simulink model "lab04z2_sch"  (Simulink 10.3)
settings: Solver=ode3  StartTime=0.0  StopTime=10  FixedStep=0.001  RelTol=1e-3  EnableMultiTasking=on
InitFcn:
  | % Parametry obiektu
  | R = 3;
  | L = 0.05;
  | kfi = 2.23;
  | J = 0.11;
values from neighbouring files (symbols this model uses):
  ki = 1    [lab04z1.m]
  Kx = acker(A, B, [-wc, -wc])    [lab04z1.m]
  Lo = acker(A', C', [-w0, -w0])    [lab04z1.m]
undefined symbols (not defined in the file or in its folder): regStan
settings Model: Creator=Jacek  LastModifiedBy=AgraWoodAdmin
settings DataIOCC: LimitDataPoints=on  SignalLoggingSaveFormat=Dataset
settings OptimizationCC: ExpressionDepthLimit=128
settings DebuggingCC: UnderspecifiedInitializationDetection=Simplified  MergeDetectMultiDrivingBlocksExec=error  SolverPrmCheckMsg=warning  FcnCallInpInsideContextMsg=error  StateNameClashWarn=none
settings GRTTargetCC: CombineOutputUpdateFcns=on  GRTInterface=off
settings ConfigComp: CovSFcnEnable=off

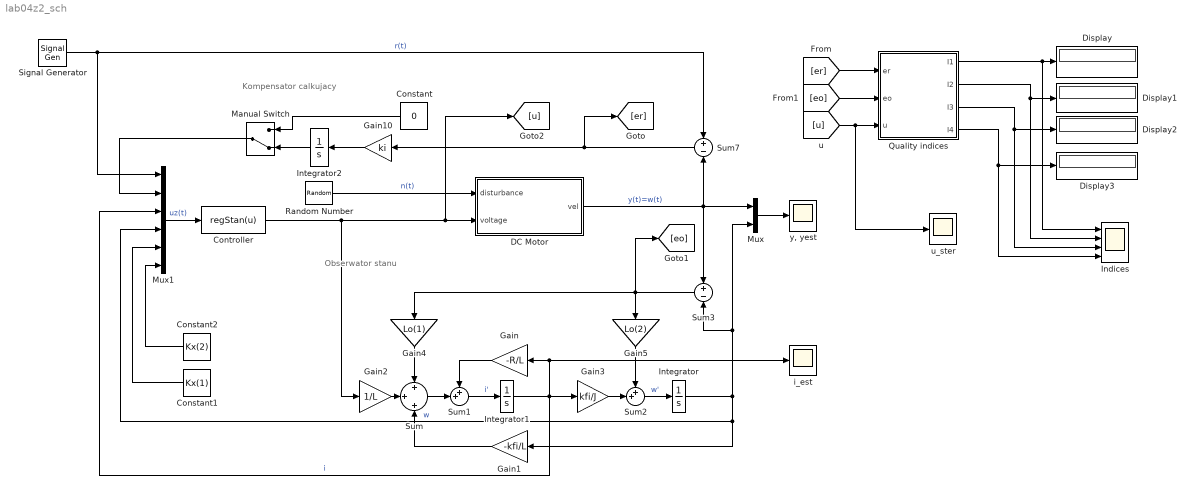
== system lab04z2_sch ==
  note: Kompensator calkujacy
  note: Obserwator stanu
  Constant : Constant  Value=0
  Constant1 : Constant  Value=Kx(1)
  Constant2 : Constant  Value=Kx(2)
  Controller : MATLABFcn  MATLABFcn=regStan(u)  OutputDimensions=1
  DC Motor : Subsystem
  Display{,1..3} (4 alike) : Display
  Gain : Gain  Gain=-R/L
  Gain1 : Gain  Gain=-kfi/L
  Gain10 : Gain  Gain=ki
  Gain2 : Gain  Gain=1/L
  Gain3 : Gain  Gain=kfi/J
  Gain4 : Gain  Gain=Lo(1)
  Gain5 : Gain  Gain=Lo(2)
  Indices : Scope  NumInputPorts=4
  Integrator : Integrator  InitialCondition=40
  Integrator1 : Integrator  InitialCondition=20
  Integrator2 : Integrator
  Manual Switch : ManualSwitch  CurrentSetting=0
  Mux : Mux  Inputs=2
  Mux1 : Mux  Inputs=6
  Quality indices : Subsystem
  Random Number : RandomNumber  Variance=10
  Signal Generator : SignalGenerator  WaveForm=square  Amplitude=200  Frequency=0.5
  Sum : Sum  Inputs=+|+|+
  Sum1 : Sum  Inputs=++|
  Sum2 : Sum  Inputs=++|
  Sum3 : Sum  Inputs=+|-
  Sum7 : Sum  Inputs=+|-
  i_est : Scope
  u_ster : Scope
  "y, yest" : Scope
  wires:
  Random Number/1 -> DC Motor/1(disturbance)  "n(t)"
  Mux1/1 -> Controller/1  "uz(t)"
  DC Motor/1(vel) -> Sum3/1, Sum7/2, Mux/1  "y(t)=w(t)"
  Gain2/1 -> Sum/2
  Sum1/1 -> Integrator1/1  "i'"
  Gain/1 -> Sum1/1
  Sum/1 -> Sum1/2
  Gain1/1 -> Sum/3
  Sum2/1 -> Integrator/1  "w'"
  Gain3/1 -> Sum2/2
  Sum3/1 -> [eo], Gain5/1, Gain4/1
  Gain5/1 -> Sum2/1
  Gain4/1 -> Sum/1
  Mux/1 -> "y, yest"/1
  Integrator/1 -> Mux1/4, Gain1/1, Sum3/2, Mux/2  "w"
  Integrator1/1 -> i_est/1, Gain/1, Mux1/3, Gain3/1  "i"
  Signal Generator/1 -> Mux1/1, Sum7/1  "r(t)"
  Integrator2/1 -> Manual Switch/2
  Sum7/1 -> [er], Gain10/1
  Gain10/1 -> Integrator2/1
  Manual Switch/1 -> Mux1/2
  Constant/1 -> Manual Switch/1
  Quality indices/4(I4) -> Indices/4, Display3/1
  Quality indices/1(I1) -> Indices/1, Display/1
  Quality indices/2(I2) -> Display1/1, Indices/2
  Quality indices/3(I3) -> Display2/1, Indices/3
  [er] -> Quality indices/1(er)
  [eo] -> Quality indices/2(eo)
  [u] -> u_ster/1, Quality indices/3(u)
  Constant2/1 -> Mux1/6
  Constant1/1 -> Mux1/5
  Controller/1 -> Gain2/1, [u], DC Motor/2(voltage)

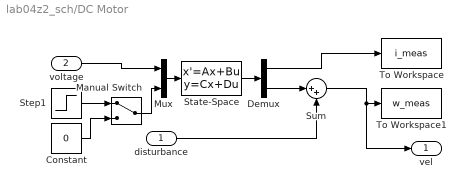
== system lab04z2_sch/DC Motor ==
  disturbance : Inport
  voltage : Inport  Port=2
  Constant : Constant  Value=0
  Demux : Demux  Outputs=2
  Manual Switch : ManualSwitch
  Mux : Mux  Inputs=2
  State-Space : StateSpace  A=[-3/0.05, -2.23/0.05; 2.23/0.11, 0]  B=[1/0.05 0; 0 -1/0.11]  C=[1 0;0 1]  D=[0 0; 0 0]  InitialCondition=[0 ;40]
  Step1 : Step  Time=0.5  After=44.6*1  SampleTime=0
  Sum : Sum  Inputs=|++
  To Workspace : ToWorkspace  VariableName=i_meas  SampleTime=-1
  To Workspace1 : ToWorkspace  VariableName=w_meas  SampleTime=-1
  vel : Outport  VectorParamsAs1DForOutWhenUnconnected=off
  wires:
  Mux/1 -> State-Space/1
  voltage/1 -> Mux/1
  Step1/1 -> Manual Switch/1
  State-Space/1 -> Demux/1
  Demux/1 -> To Workspace/1
  disturbance/1 -> Sum/2
  Sum/1 -> vel/1, To Workspace1/1
  Demux/2 -> Sum/1
  Manual Switch/1 -> Mux/2
  Constant/1 -> Manual Switch/2

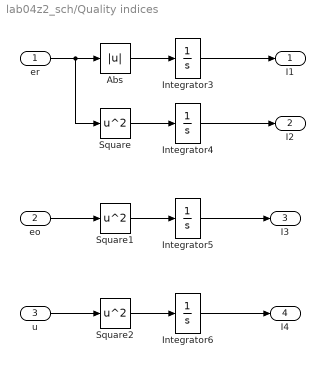
== system lab04z2_sch/Quality indices ==
  er : Inport
  eo : Inport  Port=2
  u : Inport  Port=3
  Abs : Abs
  Integrator{3..6} (4 alike) : Integrator
  Square : Math  Operator=square  SignedPower=on  RndMeth=Zero  SaturateOnIntegerOverflow=on
  Square1 : Math  Operator=square  SignedPower=on  RndMeth=Zero  SaturateOnIntegerOverflow=on
  Square2 : Math  Operator=square  SignedPower=on  RndMeth=Zero  SaturateOnIntegerOverflow=on
  I1 : Outport  VectorParamsAs1DForOutWhenUnconnected=off
  I2 : Outport  Port=2  VectorParamsAs1DForOutWhenUnconnected=off
  I3 : Outport  Port=3  VectorParamsAs1DForOutWhenUnconnected=off
  I4 : Outport  Port=4  VectorParamsAs1DForOutWhenUnconnected=off
  wires:
  eo/1 -> Square1/1
  Square2/1 -> Integrator6/1
  Integrator6/1 -> I4/1
  u/1 -> Square2/1
  er/1 -> Abs/1, Square/1
  Integrator4/1 -> I2/1
  Square1/1 -> Integrator5/1
  Integrator5/1 -> I3/1
  Abs/1 -> Integrator3/1
  Integrator3/1 -> I1/1
  Square/1 -> Integrator4/1
